simulink model "simple"  (R2013a)
settings: Solver=ode45  StartTime=0.0  StopTime=5.0  RelTol=1e-3
StartFcn:
  | evalin('base', 'initEnv');
settings Model: Creator=Sunil  LastModifiedBy=Sunil

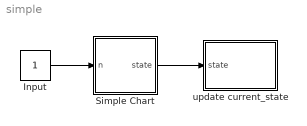
== system simple ==
  "Input " : Constant
  Simple Chart : Stateflow chart  TreatAsAtomicUnit=on
  update current_state : MATLAB Function  TreatAsAtomicUnit=on
  wires:
  "Input "/1 -> Simple Chart/1(n)
  Simple Chart/1(state) -> update current_state/1(state)

== stateflow chart simple/Simple Chart ==
  state start
    en: x = n;
    y = 1;
    du: x = x + 1;
    y = y + 1;
    ex:
  state C
    en:
    du:
    ex: y = y + 5;
  state A
    en: x = x + 2;
    y = y + 1;
    du:
    ex:
  A -> C : [x ~= 10]/{x = x + 1; }
  (default) -> start : []/{}
  start -> C : [x < 5]/{x = x + 1;}
  C -> A : [x < 10]/{x = x - 1;}
  data: n input; x local double; y local double; state output Enum: state_name

== matlab function simple/update current_state ==
  data: state input
function fcn(state)
%#codegen
% Sets the 'new_state' variable in the 
% base workspace to the Active State Output from Stateflow Chart 
% 'Simple Chart'
% See Active State Output in Stateflow documentation for details

    coder.extrinsic('assignin');
    assignin('base', 'new_state', state);
